simulink model "variable_stiffness_Based_Position"  (R2018b)
settings: Solver=FixedStepAuto  StartTime=0.0  StopTime=1  FixedStep=0.0005  MaxStep=0.002  MinStep=0.001  RelTol=1e-3
model workspace: external: MATLAB File G:\MATLAB\SCARA\SCARA_Robot_DataFile.m (data not in the file)
values from neighbouring files (symbols this model uses):
  Ball = struct    [SCARA_Robot_DataFile.m]
  coff = [1 40 400]    [SCARA_Robot_DataFile.m]
  Plane = struct    [SCARA_Robot_DataFile.m]
  smiData = struct    [SCARA_Robot_DataFile.m]
undefined symbols (not defined in the file or in its folder): sigbuilder_block, X, Y, Z
libraries: sm_lib x81, nesl_utility x44, robotmaniplib x9, Contact_Forces_Lib x3, Parts_Lib x2, cstblocks x1, simulink x1
(part 1 of 2)
settings Model: Creator=wqq  LastModifiedBy=wqq
settings SolverCC: InitialStep=0.001  ZeroCrossAlgorithm=Adaptive
settings DebuggingCC: IgnoredZcDiagnostic=none

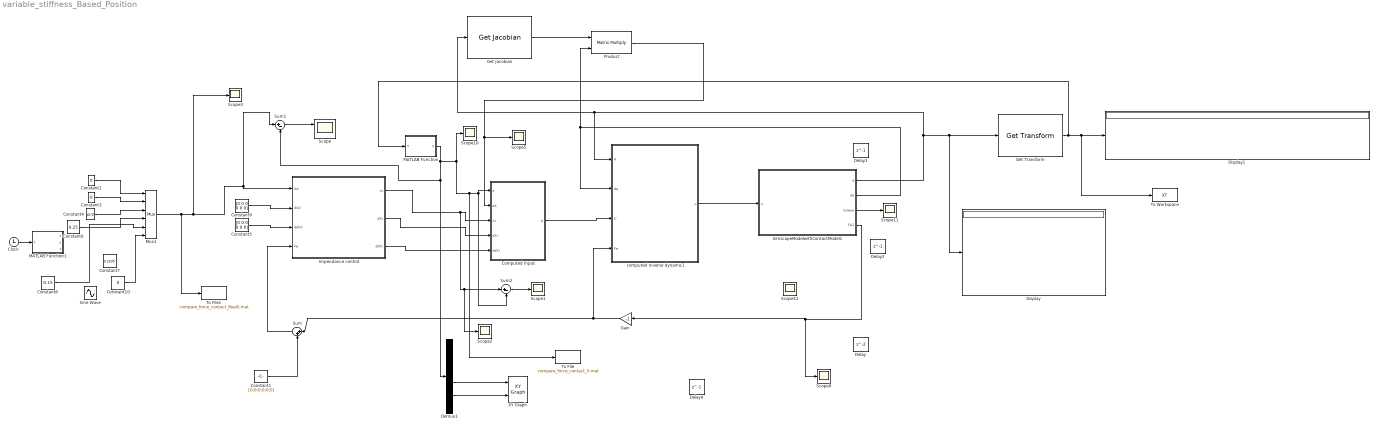
== system variable_stiffness_Based_Position ==
  " Computed Input" : Subsystem
  Clock : Clock
  Constant1 : Constant  Value=[0;0;0;0;0;0]  VectorParams1D=off
  Constant10 : Constant  Value=0
  Constant2 : Constant  Value=0
  Constant3 : Constant  Value=0
  Constant4 : Constant  Value=pi/2
  Constant5 : Constant  Value=[0 0 0 0 0 0]  VectorParams1D=off
  Constant6 : Constant  Value=0.25
  Constant7 : Constant  Value=0.2235
  Constant8 : Constant  Value=0.15
  Constant9 : Constant  Value=[0 0 0 0 0 0]  VectorParams1D=off
  Delay : Delay
  Delay1 : Delay  DelayLength=1  InitialCondition=[0;pi/2;0;0]
  Delay2 : Delay  DelayLength=1  InitialCondition=[0;0;0;0]
  Delay4 : Delay  DelayLength=1  InitialCondition=[0;0;0;0;0;0]
  Demux1 : Demux  Outputs=6
  Display : Display
  Display1 : Display
  Gain : Gain  Gain=-1
  Get Jacobian : robotmaniplib/Get Jacobian  RigidBodyTree=SCARA_Robot  EndEffector=Body5
      settings: SourceProductName=Robotics System Toolbox
  Get Transform : robotmaniplib/Get Transform  RigidBodyTree=SCARA_Robot  SourceBody=Body5  TargetBody=Body7
      settings: SourceProductName=Robotics System Toolbox
  Impendance control : Subsystem
  MATLAB Function : MATLAB Function  TreatAsAtomicUnit=on
  MATLAB Function1 : MATLAB Function  TreatAsAtomicUnit=on
  Mux1 : Mux  Inputs=6
  Product : Product  Multiplication=Matrix(*)
  Scope : Scope  NumInputPorts=2
  Scope{1..3,5,9..12} (8 alike) : Scope
  SimscapeModelwithContactModel1 : Subsystem
      mask Display: image('SCARA_picture.png');
  Sine Wave : Sin  Amplitude=0.5  Bias=0.2235  Frequency=3  SampleTime=0
  Sum : Sum  Inputs=|++
  Sum1 : Sum  Inputs=|+-
  Sum2 : Sum  Inputs=|+-
  To File : ToFile  Filename=compare_force_contact_X.mat  MatrixName=X  SaveFormat=Timeseries
  To File1 : ToFile  Filename=compare_force_contact_RealX.mat  MatrixName=RealX  SaveFormat=Timeseries
  To Workspace : ToWorkspace  VariableName=XT  SaveFormat=Timeseries  SampleTime=-1
  XY Graph : simulink/Sinks/XY Graph  xmin=-0.4  xmax=0.4  ymin=-0.4  ymax=0.4  st=-1
  computed Inverse dynamic1 : Subsystem
  wires:
  SimscapeModelwithContactModel1/3(torque) -> Scope11/1
  Demux1/4 -> XY Graph/1
  Demux1/5 -> XY Graph/2
  Product/1 -> Scope5/1, " Computed Input"/2(dX)
  Get Jacobian/1 -> Product/1
  Constant3/1 -> Mux1/2
  Constant2/1 -> Mux1/1
  " Computed Input"/1(U) -> computed Inverse dynamic1/3(U)
  Clock/1 -> MATLAB Function1/1(t)
  Get Transform/1 -> MATLAB Function/1(T), To Workspace/1, Display1/1
  MATLAB Function/1(X) -> Sum1/2, Demux1/1, Scope10/1, To File/1, " Computed Input"/1(X), Sum2/2
  Constant4/1 -> Mux1/3
  Impendance control/1(Xr) -> Scope2/1, Sum2/1, " Computed Input"/3(Xr)
  Impendance control/2(dXr) -> " Computed Input"/4(dXr)
  Mux1/1 -> To File1/1, Scope3/1, Sum1/1, Impendance control/1(Xd)
  Constant9/1 -> Impendance control/2(dXd)
  Constant5/1 -> Impendance control/3(ddXd)
  Impendance control/3(ddXr) -> " Computed Input"/5(ddXr)
  Sum/1 -> Impendance control/4(Fe)
  Constant1/1 -> Sum/2
  SimscapeModelwithContactModel1/4(Fe1) -> Gain/1, Scope9/1
  SimscapeModelwithContactModel1/2(dq) -> computed Inverse dynamic1/2(dq), Product/2
  SimscapeModelwithContactModel1/1(q) -> Display/1, Get Transform/1, computed Inverse dynamic1/1(q), Get Jacobian/1
  Sum1/1 -> Scope/1
  Sum2/1 -> Scope1/1
  Gain/1 -> computed Inverse dynamic1/4(Fe), Sum/1
  Constant6/1 -> Mux1/4
  Constant8/1 -> Mux1/5
  Constant10/1 -> Mux1/6
  computed Inverse dynamic1/1(u) -> SimscapeModelwithContactModel1/1(u)

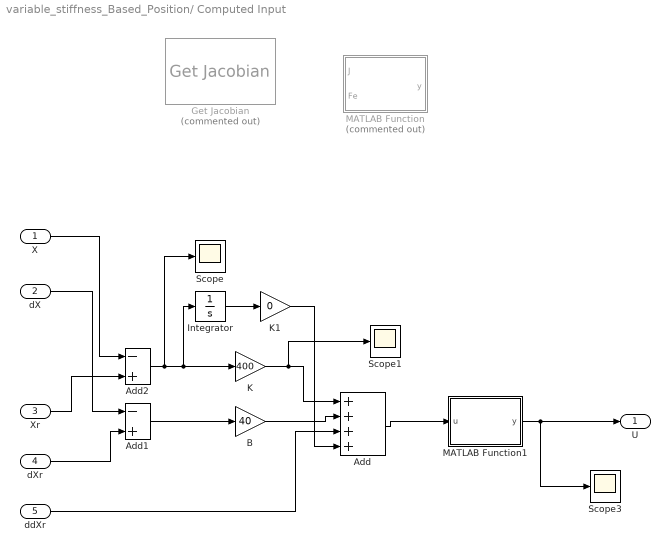
== system variable_stiffness_Based_Position/ Computed Input ==
  X : Inport
  dX : Inport  Port=2
  Xr : Inport  Port=3
  dXr : Inport  Port=4
  ddXr : Inport  Port=5
  Add : Sum  Inputs=++++
  Add1 : Sum  Inputs=-+
  Add2 : Sum  Inputs=-+
  B : Gain  Gain=40
  Get Jacobian : robotmaniplib/Get Jacobian  Commented=on  RigidBodyTree=SCARA_Robot  EndEffector=Body5
      settings: SourceProductName=Robotics System Toolbox
  Integrator : Integrator
  K : Gain  Gain=400
  K1 : Gain  Gain=0
  MATLAB Function : MATLAB Function  Commented=on  TreatAsAtomicUnit=on
  MATLAB Function1 : MATLAB Function  TreatAsAtomicUnit=on
  Scope : Scope
  Scope1 : Scope
  Scope3 : Scope
  U : Outport
  wires:
  ddXr/1 -> Add/3
  dXr/1 -> Add1/2
  dX/1 -> Add1/1
  B/1 -> Add/2
  Xr/1 -> Add2/2
  K/1 -> Scope1/1, Add/1
  Add/1 -> MATLAB Function1/1(u)
  X/1 -> Add2/1
  Add2/1 -> Integrator/1, K/1, Scope/1
  Add1/1 -> B/1
  MATLAB Function1/1(y) -> U/1, Scope3/1
  Integrator/1 -> K1/1
  K1/1 -> Add/4

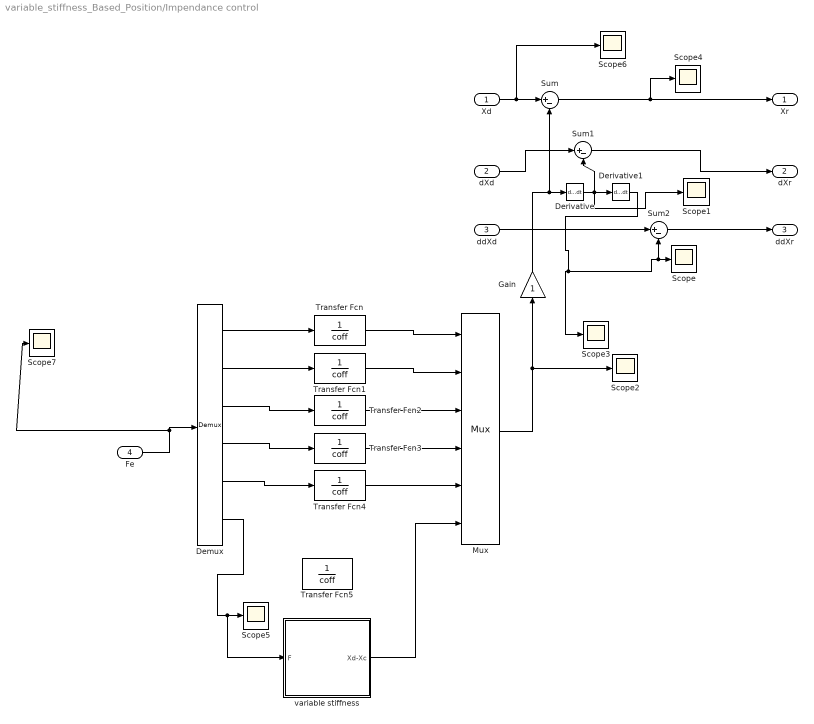
== system variable_stiffness_Based_Position/Impendance control ==
  Xd : Inport
  dXd : Inport  Port=2
  ddXd : Inport  Port=3
  Fe : Inport  Port=4
  Demux : Demux  Outputs=6
  Derivative : Derivative
  Derivative1 : Derivative
  Gain : Gain
  Mux : Mux  Inputs=6
  Scope{,1..7} (8 alike) : Scope
  Sum : Sum  Inputs=|+-
  Sum1 : Sum  Inputs=|+-
  Sum2 : Sum  Inputs=|+-
  Transfer Fcn{,1..5} (6 alike) : TransferFcn  Denominator=coff
  variable stiffness : Subsystem
  Xr : Outport
  dXr : Outport  Port=2
  ddXr : Outport  Port=3
  wires:
  Xd/1 -> Scope6/1, Sum/1
  Sum/1 -> Scope4/1, Xr/1
  dXd/1 -> Sum1/1
  Sum1/1 -> dXr/1
  ddXd/1 -> Sum2/1
  Derivative/1 -> Scope1/1, Derivative1/1, Sum1/2
  Sum2/1 -> ddXr/1
  Demux/1 -> Transfer Fcn/1
  Demux/2 -> Transfer Fcn1/1
  Demux/3 -> Transfer Fcn2/1
  Demux/4 -> Transfer Fcn3/1
  Demux/5 -> Transfer Fcn4/1
  Transfer Fcn4/1 -> Mux/5
  Transfer Fcn3/1 -> Mux/4
  Transfer Fcn2/1 -> Mux/3
  Transfer Fcn1/1 -> Mux/2
  Transfer Fcn/1 -> Mux/1
  Mux/1 -> Scope2/1, Gain/1
  Gain/1 -> Sum/2, Derivative/1
  Fe/1 -> Scope7/1, Demux/1
  Derivative1/1 -> Sum2/2, Scope/1, Scope3/1
  Demux/6 -> variable stiffness/1(F), Scope5/1
  variable stiffness/1(Xd-Xc) -> Mux/6

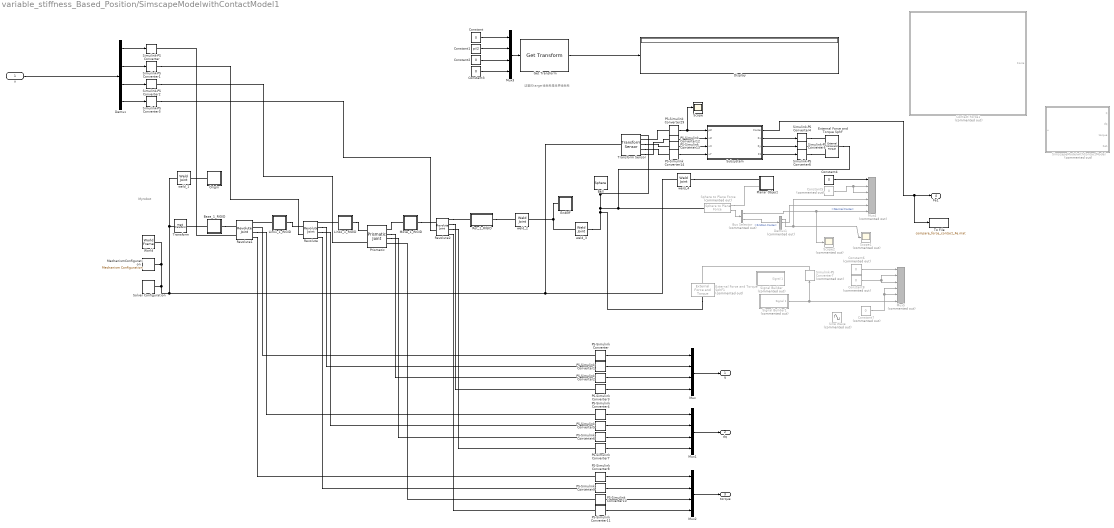
== system variable_stiffness_Based_Position/SimscapeModelwithContactModel1 ==
  note: 这里的target坐标系是世界坐标系
  note: Myrobot
  u : Inport
  Ball : Parts_Lib/Sphere  Tag=CustomStyle  sph_radius=Ball.radius  sph_density=Ball.density  sph_color=red  sph_opacity=1  mark_type=Rings on center planes  arc_width=[40 50]  arc_angle=60  ring_width=5  ring_irad=0.95  mark_color=axes  mark_opacity_x=1  mark_opacity_y=1  mark_opacity_z=1  mark_opacity=1  ring_opacity=0  arc_opacity=0  arc_extr_data=0
  Base_1_RIGID : Subsystem
  Bus Selector : BusSelector  Commented=on  OutputSignals=Normal Force,Friction Force
  Constant{,2..4} (4 alike) : Constant  Value=0
  Constant1 : Constant  Value=pi/2
  Constant{5..8} (4 alike) : Constant  Commented=on  Value=0
  Contact Force1 : Subsystem  Commented=on
  Demux : Demux
  Demux1 : Demux  Commented=on  Outputs=3
  Display : Display
  EndEff : Subsystem
  External Force and Torque SphF : sm_lib/Forces and Torques/External Force and Torque  ForceResolutionFrame=AttachedFrame  EnableForceX=on  EnableForceY=on  EnableForceZ=on  EnableForce=off  TorqueResolutionFrame=AttachedFrame  EnableTorqueX=off  EnableTorqueY=off  EnableTorqueZ=off  EnableTorque=off
  External Force and Torque SphF1 : sm_lib/Forces and Torques/External Force and Torque  Commented=on  ForceResolutionFrame=World  EnableForceX=off  EnableForceY=off  EnableForceZ=on  EnableForce=off  TorqueResolutionFrame=AttachedFrame  EnableTorqueX=off  EnableTorqueY=off  EnableTorqueZ=off  EnableTorque=off
  Get Transform : robotmaniplib/Get Transform  RigidBodyTree=SCARA_Robot  SourceBody=Body5  TargetBody=Body7
      settings: SourceProductName=Robotics System Toolbox
  Link1_1_RIGID : Subsystem
  Link2_1_RIGID : Subsystem
  MechanismConfiguration : sm_lib/Utilities/Mechanism Configuration  UniformGravity=Constant  GravityVector=[0 0 -9.80665]  GravityUnits=m/s^2  LinearizationDelta=0.001
  Move_1_RIGID : Subsystem
  Mux{,1..3} (4 alike) : Mux
  Mux4 : Mux  Commented=on  Inputs=6
  Mux5 : Mux  Commented=on  Inputs=6
  Origin : Subsystem
  PS-Simulink Converter{,1..14,29} (16 alike) : nesl_utility/PS-Simulink Converter  PhysicalDomain=network_engine_domain  SubClassName=ps_output  LeftPortType=input  RightPortType=output  PseudoPeriodic=off  Frequencies=[]  Unit=1  AffineConversion=off
  Planar Object : Subsystem
  Prismatic : sm_lib/Joints/Prismatic Joint  SenseConstraintForce=off  SenseConstraintForceX=off  SenseConstraintForceY=off  SenseConstraintForceZ=off  SenseConstraintTorque=off  SenseConstraintTorqueX=off  SenseConstraintTorqueY=off  SenseConstraintTorqueZ=off  SenseTotalForce=off  SenseTotalForceX=off  SenseTotalForceY=off  SenseTotalForceZ=off  SenseTotalTorque=off  SenseTotalTorqueX=off  SenseTotalTorqueY=off  SenseTotalTorqueZ=off  CompositeWrenchDir=FollowerOnBase  CompositeWrenchFrame=BaseFrame  EquilibriumPosition=0  EquilibriumPositionUnits=m  SpringStiffness=0  SpringStiffnessUnits=N/m  DampingCoefficient=0  DampingCoefficientUnits=N/(m/s)  TorqueActuationMode=InputTorque  MotionActuationMode=ComputedMotion  SensePosition=on  SenseVelocity=on  SenseAcceleration=off  SenseTorqueForce=on  PositionTargetSpecify=on  PositionTargetPriority=High  PositionTargetValue=smiData.PrismaticJoint(1).Pz.Pos  PositionTargetValueUnits=m  VelocityTargetSpecify=off  VelocityTargetPriority=High  VelocityTargetValue=0  VelocityTargetValueUnits=m/s
  Revolute : sm_lib/Joints/Revolute Joint  SenseConstraintForce=off  SenseConstraintForceX=off  SenseConstraintForceY=off  SenseConstraintForceZ=off  SenseConstraintTorque=off  SenseConstraintTorqueX=off  SenseConstraintTorqueY=off  SenseConstraintTorqueZ=off  SenseTotalForce=off  SenseTotalForceX=off  SenseTotalForceY=off  SenseTotalForceZ=off  SenseTotalTorque=off  SenseTotalTorqueX=off  SenseTotalTorqueY=off  SenseTotalTorqueZ=off  CompositeWrenchDir=FollowerOnBase  CompositeWrenchFrame=BaseFrame  EquilibriumPosition=0  EquilibriumPositionUnits=rad  SpringStiffness=0  SpringStiffnessUnits=N*m/rad  DampingCoefficient=0  DampingCoefficientUnits=N*m/(rad/s)  TorqueActuationMode=InputTorque  MotionActuationMode=ComputedMotion  SensePosition=on  SenseVelocity=on  SenseAcceleration=off  SenseTorqueForce=on  PositionTargetSpecify=on  PositionTargetPriority=High  PositionTargetValue=smiData.RevoluteJoint(1).Rz.Pos  PositionTargetValueUnits=deg  VelocityTargetSpecify=off  VelocityTargetPriority=High  VelocityTargetValue=0  VelocityTargetValueUnits=deg/s
  Revolute1 : sm_lib/Joints/Revolute Joint  SenseConstraintForce=off  SenseConstraintForceX=off  SenseConstraintForceY=off  SenseConstraintForceZ=off  SenseConstraintTorque=off  SenseConstraintTorqueX=off  SenseConstraintTorqueY=off  SenseConstraintTorqueZ=off  SenseTotalForce=off  SenseTotalForceX=off  SenseTotalForceY=off  SenseTotalForceZ=off  SenseTotalTorque=off  SenseTotalTorqueX=off  SenseTotalTorqueY=off  SenseTotalTorqueZ=off  CompositeWrenchDir=FollowerOnBase  CompositeWrenchFrame=BaseFrame  EquilibriumPosition=0  EquilibriumPositionUnits=rad  SpringStiffness=0  SpringStiffnessUnits=N*m/rad  DampingCoefficient=0  DampingCoefficientUnits=N*m/(rad/s)  TorqueActuationMode=InputTorque  MotionActuationMode=ComputedMotion  SensePosition=on  SenseVelocity=on  SenseAcceleration=off  SenseTorqueForce=on  PositionTargetSpecify=on  PositionTargetPriority=High  PositionTargetValue=smiData.RevoluteJoint(2).Rz.Pos  PositionTargetValueUnits=deg  VelocityTargetSpecify=off  VelocityTargetPriority=High  VelocityTargetValue=0  VelocityTargetValueUnits=deg/s
  Revolute2 : sm_lib/Joints/Revolute Joint  SenseConstraintForce=off  SenseConstraintForceX=off  SenseConstraintForceY=off  SenseConstraintForceZ=off  SenseConstraintTorque=off  SenseConstraintTorqueX=off  SenseConstraintTorqueY=off  SenseConstraintTorqueZ=off  SenseTotalForce=off  SenseTotalForceX=off  SenseTotalForceY=off  SenseTotalForceZ=off  SenseTotalTorque=off  SenseTotalTorqueX=off  SenseTotalTorqueY=off  SenseTotalTorqueZ=off  CompositeWrenchDir=FollowerOnBase  CompositeWrenchFrame=BaseFrame  EquilibriumPosition=0  EquilibriumPositionUnits=rad  SpringStiffness=0  SpringStiffnessUnits=N*m/rad  DampingCoefficient=0  DampingCoefficientUnits=N*m/(rad/s)  TorqueActuationMode=InputTorque  MotionActuationMode=ComputedMotion  SensePosition=on  SenseVelocity=on  SenseAcceleration=off  SenseTorqueForce=on  PositionTargetSpecify=on  PositionTargetPriority=High  PositionTargetValue=smiData.RevoluteJoint(3).Rz.Pos  PositionTargetValueUnits=deg  VelocityTargetSpecify=off  VelocityTargetPriority=High  VelocityTargetValue=0  VelocityTargetValueUnits=deg/s
  Rot_1_RIGID : Subsystem
  Scope : Scope
  Scope1 : Scope  Commented=on
  Scope2 : Scope  Commented=on
  Signal Builder : Subsystem  Tag=STV Subsys  Commented=on  LoadFcn=sigbuilder_block('load');  StartFcn=sigbuilder_block('start');  StopFcn=sigbuilder_block('stop');  ClipboardFcn=sigbuilder_block('clipboard');  mask(Sigbuilder block){tuvar=[0:10]}
      mask help: Simulink:masks:SigbuilderBlock_MD
      mask init:
      | if ~strcmp(get_param(bdroot(gcbh),'SimulationStatus'),'stopped') tuvar = sigbuilder_block('maskInit'); end
      settings: CopyFcn=sigbuilder_block('copy');  DeleteFcn=sigbuilder_block('delete');  ModelCloseFcn=sigbuilder_block('modelClose');  PreSaveFcn=sigbuilder_block('preSave');  PauseFcn=sigbuilder_block('pause');  ContinueFcn=sigbuilder_block('continue');  NameChangeFcn=sigbuilder_block('namechange');  OpenFcn=sigbuilder_block('open',[437.6 199.2 550.4 400 ]);  CloseFcn=sigbuilder_block('close');
      mask Display: plot(0, 0, 100, 100,[2, 2, 32, 32, 2], [68, 8, 8, 68, 68],[32, 2], [38, 38], [32, 19, 2],[53, 60, 44], [32, 17, 17, 2],[16, 16, 31, 31]);txt = getActiveGroup(gcbh);text(2, 100, txt,'verticalAlignment', 'top');
  Signal Builder1 : Subsystem  Tag=STV Subsys  Commented=on  LoadFcn=sigbuilder_block('load');  StartFcn=sigbuilder_block('start');  StopFcn=sigbuilder_block('stop');  ClipboardFcn=sigbuilder_block('clipboard');  mask(Sigbuilder block){tuvar=[0:10]}
      mask help: Simulink:masks:SigbuilderBlock_MD
      mask init:
      | if ~strcmp(get_param(bdroot(gcbh),'SimulationStatus'),'stopped') tuvar = sigbuilder_block('maskInit'); end
      settings: CopyFcn=sigbuilder_block('copy');  DeleteFcn=sigbuilder_block('delete');  ModelCloseFcn=sigbuilder_block('modelClose');  PreSaveFcn=sigbuilder_block('preSave');  PauseFcn=sigbuilder_block('pause');  ContinueFcn=sigbuilder_block('continue');  NameChangeFcn=sigbuilder_block('namechange');  OpenFcn=sigbuilder_block('open',[437.6 199.2 550.4 400 ]);  CloseFcn=sigbuilder_block('close');
      mask Display: plot(0, 0, 100, 100,[2, 2, 32, 32, 2], [68, 8, 8, 68, 68],[32, 2], [38, 38], [32, 19, 2],[53, 60, 44], [32, 17, 17, 2],[16, 16, 31, 31]);txt = getActiveGroup(gcbh);text(2, 100, txt,'verticalAlignment', 'top');
  SimscapeModelwithContactModel : Subsystem  Commented=on
  Simulink-PS Converter{,1..6} (7 alike) : nesl_utility/Simulink-PS Converter  PhysicalDomain=network_engine_domain  SubClassName=ps_input  LeftPortType=input  RightPortType=output  PseudoPeriodic=off  Frequencies=[]  NoiseDistribution=none  NoiseParameters=[]  Unit=1  AffineConversion=off  FilteringAndDerivatives=provide  SimscapeFilterOrder=1  InputFilterTimeConstant=0.001  UdotUserProvided=0
  Simulink-PS Converter7 : nesl_utility/Simulink-PS Converter  Commented=on  PhysicalDomain=network_engine_domain  SubClassName=ps_input  LeftPortType=input  RightPortType=output  PseudoPeriodic=off  Frequencies=[]  NoiseDistribution=none  NoiseParameters=[]  Unit=1  AffineConversion=off  FilteringAndDerivatives=provide  SimscapeFilterOrder=1  InputFilterTimeConstant=0.001  UdotUserProvided=0
  Sine Wave : Sin  Commented=on  Amplitude=20  SampleTime=0
  Solver Configuration : nesl_utility/Solver Configuration  PhysicalDomain=network_engine_domain  SubClassName=solver  LeftPortType=input  RightPortType=generic  Tones=[]  Harmonics=[]  SimulateNoise=off  Profile=off  UseLocalSampling=off  EnableSwitchedLinearOptims=on  FrequencyDomain=off  UseCCode=off  RelTol=0.001  AbsTol=1e-06  MinStep=1e-09  ToWorkspace=off  RevertToSquareIcSolve=off  NumHomotopyIterations=100  PhasorMode=off  PhasorModeNumHarmonics=1  DoDC=off  ResidualTolerance=1e-09  UseLocalSolver=off  LocalSolverChoice=NE_BACKWARD_EULER_ADVANCER  LocalSolverSampleTime=0.001  DoFixedCost=off  MaxNonlinIter=3  MaxModeIter=2  LinearAlgebra=auto  EquationFormulation=NE_TIME_EF  DelaysMemoryBudget=1024  AutomaticFiltering=on  FilteringTimeConstant=0.001  PartitionStorageMethod=AS_NEEDED  PartitionMemoryBudget=1024
  Sphere to Plane Force : Contact_Forces_Lib/3D/Sphere to Plane Force  Commented=on  sphere_rad=0.03  plane_lenx=1  plane_leny=1  plane_depth=0.1/2  force_law=Linear  k_contact=1e5  b_contact=1e2  pen_full_damp_F=1e-4  pen_exponent=1  custom_param_1=1  custom_param_2=1  friction_law=Stick-Slip Continuous  mu_kinetic=0.5  mu_static=0.7  v_thr=0.001  vis_on=off  vis_opc_en=0  vis_len_plaBz=0.005  vis_clr=[0.9 0.2 0.2]  vis_opc=0.7
  Subsystem : Subsystem
  To File : ToFile  Filename=compare_force_contact_Fe.mat  MatrixName=Fe  SaveFormat=Timeseries
  Transform : sm_lib/Frames and Transforms/Rigid Transform  TranslationMethod=Cartesian  TranslationStandardOffset=0  TranslationLengthUnit=mm  TranslationStandardAxis=+Z  TranslationCartesianOffset=smiData.RigidTransform(9).translation  TranslationROffset=0  TranslationROffsetUnits=m  TranslationZOffset=0  TranslationZOffsetUnits=m  TranslationThetaOffset=0  TranslationThetaOffsetUnits=deg  RotationMethod=ArbitraryAxis  RotationAngleUnits=rad  RotationStandardAxis=+Z  RotationAngle=smiData.RigidTransform(9).angle  RotationArbitraryAxis=smiData.RigidTransform(9).axis  FollAlignAxisA=+X  BaseAlignAxisA=+Y  FollAlignAxisB=+Y  BaseAlignAxisB=+Z  RotationSequenceAxes=FollowerAxes  RotationSequence=XYX  RotationSequenceAngles=[0 0 0]  RotationSequenceAnglesUnits=deg  RotationMatrix=[1 0 0; 0 1 0; 0 0 1]
  Transform Sensor : sm_lib/Frames and Transforms/Transform Sensor  MeasurementFrame=World  SenseAngle=off  SenseAxis=off  SenseAngle1=off  SenseAngle2=off  SenseAngle3=off  SenseQ=off  SenseR=off  SenseOmegaX=off  SenseOmegaY=off  SenseOmegaZ=off  SenseOmega1=off  SenseOmega2=off  SenseOmega3=off  SenseQDot=off  SenseRDot=off  SenseAlphaX=off  SenseAlphaY=off  SenseAlphaZ=off  SenseAlpha1=off  SenseAlpha2=off  SenseAlpha3=off  SenseQDDot=off  SenseRDDot=off  SenseX=off  SenseY=off  SenseZ=on  SenseRad=off  SenseAzim=off  SenseDist=off  SenseInc=off  SenseXDot=on  SenseYDot=on  SenseZDot=on  SenseRadDot=off  SenseAzimDot=off  SenseDistDot=off  SenseIncDot=off  SenseXDDot=off  SenseYDDot=off  SenseZDDot=off  SenseRadDDot=off  SenseAzimDDot=off  SenseDistDDot=off  SenseIncDDot=off
  World : sm_lib/Frames and Transforms/World Frame
  weld_{1..4} (4 alike) : sm_lib/Joints/Weld Joint  SenseConstraintForce=off  SenseConstraintForceX=off  SenseConstraintForceY=off  SenseConstraintForceZ=off  SenseConstraintTorque=off  SenseConstraintTorqueX=off  SenseConstraintTorqueY=off  SenseConstraintTorqueZ=off  SenseTotalForce=off  SenseTotalForceX=off  SenseTotalForceY=off  SenseTotalForceZ=off  SenseTotalTorque=off  SenseTotalTorqueX=off  SenseTotalTorqueY=off  SenseTotalTorqueZ=off  CompositeWrenchDir=FollowerOnBase  CompositeWrenchFrame=BaseFrame
  q : Outport
  dq : Outport  Port=2
  torque : Outport  Port=3
  Fe1 : Outport  Port=4
  wires:
  Demux/4 -> Simulink-PS Converter3/1
  Mux1/1 -> dq/1
  PS-Simulink Converter10/1 -> Mux2/3
  PS-Simulink Converter8/1 -> Mux2/1
  Demux/1 -> Simulink-PS Converter/1
  PS-Simulink Converter11/1 -> Mux2/4
  PS-Simulink Converter5/1 -> Mux1/2
  PS-Simulink Converter/1 -> Mux/1
  Mux2/1 -> torque/1
  PS-Simulink Converter1/1 -> Mux/2
  Demux/2 -> Simulink-PS Converter1/1
  PS-Simulink Converter9/1 -> Mux2/2
  PS-Simulink Converter6/1 -> Mux1/3
  PS-Simulink Converter7/1 -> Mux1/4
  PS-Simulink Converter4/1 -> Mux1/1
  Mux/1 -> q/1
  PS-Simulink Converter2/1 -> Mux/3
  PS-Simulink Converter3/1 -> Mux/4
  Mux3/1 -> Get Transform/1
  Constant/1 -> Mux3/1
  Constant1/1 -> Mux3/2
  Constant2/1 -> Mux3/3
  Constant3/1 -> Mux3/4
  u/1 -> Demux/1
  Get Transform/1 -> Display/1
  Constant4/1 -> Mux4/1
  Constant5/1 -> Mux4/3, Mux4/2
  PS-Simulink Converter29/1 -> Scope/1, Subsystem/1(pZ)
  PS-Simulink Converter12/1 -> Subsystem/2(vZ)
  PS-Simulink Converter14/1 -> Subsystem/4(vY)
  PS-Simulink Converter13/1 -> Subsystem/3(vX)
  Demux/3 -> Simulink-PS Converter2/1
  Sphere to Plane Force/1 -> Bus Selector/1
  Bus Selector/1 -> Scope2/1, Mux4/6  "<Normal Force>"
  Bus Selector/2 -> Demux1/1  "<Friction Force>"
  Demux1/2 -> Mux4/5
  Demux1/1 -> Mux4/4, Scope1/1
  Constant8/1 -> Mux5/2, Mux5/3
  Constant6/1 -> Mux5/1
  Subsystem/2(Fx) -> Simulink-PS Converter4/1
  Subsystem/3(Fy) -> Simulink-PS Converter5/1
  Subsystem/4(Fz) -> Simulink-PS Converter6/1
  Signal Builder1/1(Signal 1) -> Simulink-PS Converter7/1, Mux5/6
  Constant7/1 -> Mux5/5, Mux5/4
  Subsystem/1(Force) -> To File/1, Fe1/1
  connections:
  Revolute2/RConn3 -- PS-Simulink Converter7/LConn1
  Revolute/RConn2 -- PS-Simulink Converter1/LConn1
  Link2_1_RIGID/LConn1 -- Revolute/RConn1
  Move_1_RIGID/LConn1 -- Prismatic/RConn1
  Link1_1_RIGID/LConn1 -- Revolute1/RConn1
  Base_1_RIGID/LConn1 -- Transform/RConn1
  Revolute2/RConn2 -- PS-Simulink Converter3/LConn1
  Revolute1/LConn2 -- Simulink-PS Converter/RConn1
  Revolute1/RConn3 -- PS-Simulink Converter4/LConn1
  Simulink-PS Converter3/RConn1 -- Revolute2/LConn2
  Revolute1/RConn4 -- PS-Simulink Converter8/LConn1
  Move_1_RIGID/RConn1 -- Revolute2/LConn1
  PS-Simulink Converter/LConn1 -- Revolute1/RConn2
  Revolute/RConn4 -- PS-Simulink Converter9/LConn1
  Link2_1_RIGID/RConn1 -- Prismatic/LConn1
  Base_1_RIGID/RConn1 -- Revolute1/LConn1
  Link1_1_RIGID/RConn1 -- Revolute/LConn1
  Revolute2/RConn1 -- Rot_1_RIGID/LConn1
  Prismatic/RConn2 -- PS-Simulink Converter2/LConn1
  Revolute2/RConn4 -- PS-Simulink Converter11/LConn1
  Simulink-PS Converter2/RConn1 -- Prismatic/LConn2
  Simulink-PS Converter1/RConn1 -- Revolute/LConn2
  Revolute/RConn3 -- PS-Simulink Converter5/LConn1
  Prismatic/RConn3 -- PS-Simulink Converter6/LConn1
  Rot_1_RIGID/RConn1 -- weld_2/LConn1
  EndEff/LConn1 -- weld_2/RConn1 -- weld_3/LConn1
  Origin/LConn1 -- weld_1/RConn1
  Ball/LConn1 -- Transform Sensor/RConn1 -- External Force and Torque SphF1/RConn1 -- weld_3/RConn1 -- External Force and Torque SphF/RConn1 -- Sphere to Plane Force/LConn1
  weld_1/LConn1 -- Transform/LConn1 -- World/RConn1 -- MechanismConfiguration/RConn1 -- Solver Configuration/RConn1 -- Transform Sensor/LConn1 -- weld_4/LConn1
  PS-Simulink Converter29/LConn1 -- Transform Sensor/RConn2
  weld_4/RConn1 -- Planar Object/LConn1
  PS-Simulink Converter10/LConn1 -- Prismatic/RConn4
  Transform Sensor/RConn3 -- PS-Simulink Converter13/LConn1
  Transform Sensor/RConn4 -- PS-Simulink Converter14/LConn1
  Transform Sensor/RConn5 -- PS-Simulink Converter12/LConn1
  Sphere to Plane Force/RConn1 -- Planar Object/LConn2
  Simulink-PS Converter4/RConn1 -- External Force and Torque SphF/LConn1
  Simulink-PS Converter5/RConn1 -- External Force and Torque SphF/LConn2
  Simulink-PS Converter6/RConn1 -- External Force and Torque SphF/LConn3
  Simulink-PS Converter7/RConn1 -- External Force and Torque SphF1/LConn1

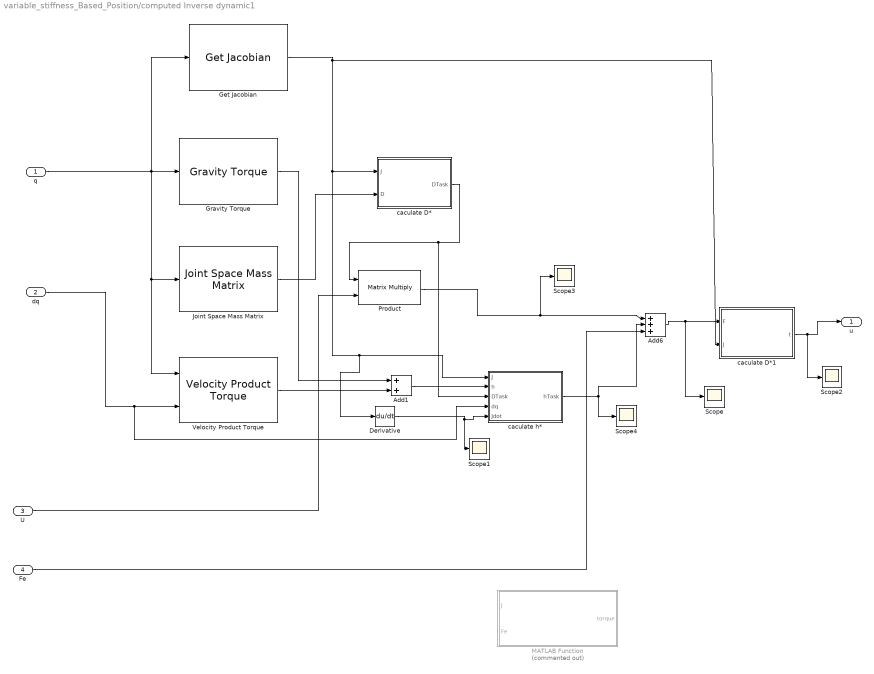
== system variable_stiffness_Based_Position/computed Inverse dynamic1 ==
  q : Inport
  dq : Inport  Port=2
  U : Inport  Port=3
  Fe : Inport  Port=4
  Add1 : Sum
  Add6 : Sum  Inputs=+++
  Derivative : Derivative
  Get Jacobian : robotmaniplib/Get Jacobian  RigidBodyTree=SCARA_Robot  EndEffector=Body5
      settings: SourceProductName=Robotics System Toolbox
  Gravity Torque : robotmaniplib/Gravity Torque  RigidBodyTree=SCARA_Robot
      settings: SourceProductName=Robotics System Toolbox
  Joint Space Mass Matrix : robotmaniplib/Joint Space Mass Matrix  RigidBodyTree=SCARA_Robot
      settings: SourceProductName=Robotics System Toolbox
  MATLAB Function : MATLAB Function  Commented=on  TreatAsAtomicUnit=on
  Product : Product  Multiplication=Matrix(*)
  Scope{,1..4} (5 alike) : Scope
  Velocity Product Torque : robotmaniplib/Velocity Product Torque  RigidBodyTree=SCARA_Robot
      settings: SourceProductName=Robotics System Toolbox
  caculate D* : MATLAB Function  TreatAsAtomicUnit=on
  caculate D*1 : MATLAB Function  TreatAsAtomicUnit=on
  caculate h* : MATLAB Function  TreatAsAtomicUnit=on
  u : Outport
  wires:
  q/1 -> Velocity Product Torque/1, Joint Space Mass Matrix/1, Get Jacobian/1, Gravity Torque/1
  Velocity Product Torque/1 -> Add1/2
  U/1 -> Product/2
  Joint Space Mass Matrix/1 -> caculate D*/2(D)
  Get Jacobian/1 -> Derivative/1, caculate h*/1(J), caculate D*/1(J), caculate D*1/2(J)
  caculate D*/1(DTask) -> caculate h*/3(DTask), Product/1
  Product/1 -> Scope3/1, Add6/1
  Gravity Torque/1 -> Add1/1
  Add1/1 -> caculate h*/2(h)
  dq/1 -> caculate h*/4(dq), Velocity Product Torque/2
  caculate D*1/1(t) -> Scope2/1, u/1
  Add6/1 -> Scope/1, caculate D*1/1(F)
  Derivative/1 -> Scope1/1, caculate h*/5(Jdot)
  caculate h*/1(hTask) -> Add6/2, Scope4/1
  Fe/1 -> Add6/3

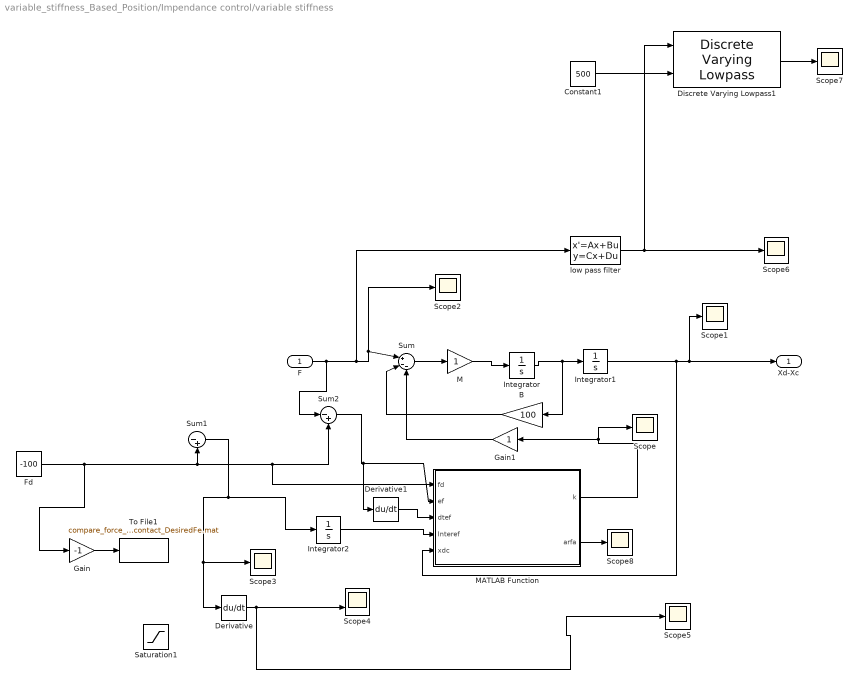
== system variable_stiffness_Based_Position/Impendance control/variable stiffness ==
  F : Inport
  B : Gain  Gain=100
  Constant1 : Constant  Value=500
  Derivative : Derivative
  Derivative1 : Derivative
  Discrete Varying Lowpass1 : cstblocks/Linear Parameter Varying/Discrete Varying Lowpass  N=1  w0=100  Ts=0.0005
      settings: SourceProductName=Control System Toolbox  SourceProductBaseCode=CT
  Fd : Constant  Value=-100
  Gain : Gain  Gain=-1
  Gain1 : Gain
  Integrator : Integrator  InitialCondition=0.0001  UpperSaturationLimit=1000  LowerSaturationLimit=-1000  IgnoreLimit=on
  Integrator1 : Integrator  InitialCondition=0.001
  Integrator2 : Integrator  UpperSaturationLimit=1000  LowerSaturationLimit=-1000  IgnoreLimit=on
  M : Gain
  MATLAB Function : MATLAB Function  TreatAsAtomicUnit=on
  Saturation1 : Saturate  UpperLimit=1000  LowerLimit=-1000
  Scope{,1..3,5..8} (8 alike) : Scope
  Scope4 : Scope  NumInputPorts=2
  Sum : Sum  Inputs=|+--
  Sum1 : Sum  Inputs=|-+
  Sum2 : Sum  Inputs=|-+
  To File1 : ToFile  Filename=compare_force_contact_DesiredFe.mat  MatrixName=DesiredFe  SaveFormat=Timeseries
  low pass filter : StateSpace  A=-100*eye(1)  B=100*eye(1)  C=eye(1)  D=zeros(1,1)  InitialCondition=zeros(1,1)
  Xd-Xc : Outport
  wires:
  Integrator/1 -> B/1, Integrator1/1
  F/1 -> Sum2/1, low pass filter/1, Scope2/1, Sum/1
  Sum/1 -> M/1
  B/1 -> Sum/2
  M/1 -> Integrator/1
  Gain1/1 -> Sum/3
  low pass filter/1 -> Discrete Varying Lowpass1/1, Scope6/1
  Integrator2/1 -> MATLAB Function/4(Interef)
  Sum1/1 -> Integrator2/1, Derivative/1, Scope3/1
  Discrete Varying Lowpass1/1 -> Scope7/1
  Constant1/1 -> Discrete Varying Lowpass1/2
  MATLAB Function/1(k) -> Gain1/1, Scope/1
  Integrator1/1 -> MATLAB Function/5(xdc), Xd-Xc/1, Scope1/1
  Derivative/1 -> Scope5/1, Scope4/2
  Gain/1 -> To File1/1
  Fd/1 -> Gain/1, MATLAB Function/1(fd), Sum2/2, Sum1/2
  MATLAB Function/2(arfa) -> Scope8/1
  Sum2/1 -> Derivative1/1, MATLAB Function/2(ef)
  Derivative1/1 -> MATLAB Function/3(dtef)

== system variable_stiffness_Based_Position/SimscapeModelwithContactModel1/Base_1_RIGID ==
  ReferenceFrame : sm_lib/Frames and Transforms/Reference Frame
  Solid : sm_lib/Body Elements/Solid  InertiaType=Custom  Mass=smiData.Solid(3).mass  MassUnits=kg  CenterOfMass=smiData.Solid(3).CoM  CenterOfMassUnits=mm  MomentsOfInertia=smiData.Solid(3).MoI  MomentsOfInertiaUnits=kg*mm^2  ProductsOfInertia=smiData.Solid(3).PoI  ProductsOfInertiaUnits=kg*mm^2  BasedOnType=Density  Density=1000  DensityUnits=kg/m^3  DoExposeReferenceFrame=off  SerializedFrames=<Frames><Frame><Id>Frame1</Id><Value><Name>F2</Name><Origin><Source>GeometricFeature</Source><FeatureName>cylindrical surface 2</FeatureName></Origin><PrimaryAxis><DefinedDirection>+Z</DefinedDirection><Source>ReferenceFrame</Source><SourceDirection>+Z</SourceDirection><FeatureName></FeatureName></PrimaryAxis><SecondaryAxis><DefinedDirection>+X</DefinedDirection><Source>ReferenceFrame</Source><SourceDirection>+X</SourceDirection><FeatureName></FeatureName></SecondaryAxis></Value></Frame></Frames>  GraphicType=FromGeometry  MarkerShape=Sphere  MarkerSize=10  GraphicVisPropType=SimpleVisualProperties  GraphicDiffuseColor=smiData.Solid(3).color  GraphicSpecularColor=[0.5 0.5 0.5 1.0]  GraphicAmbientColor=[0.15 0.15 0.15 1.0]  GraphicEmissiveColor=[0.0 0.0 0.0 1.0]  GraphicShininess=75  GraphicOpacity=smiData.Solid(3).opacity  GeometryShape=FromFile  RectangleSize=[1 1]  RectangleSizeUnits=m  BrickDimensions=[1 1 1]  BrickDimensionUnits=m  CylinderRadius=1  CylinderRadiusUnits=m  CylinderLength=1  CylinderLengthUnits=m  SphereRadius=1  SphereRadiusUnits=m  EllipsoidRadii=[1 1 1]  EllipsoidRadiiUnits=m  ExtrusionCrossSection=[1 1; -1 1; -1 -1; 1 -1]  ExtrusionCrossSectionUnits=m  ExtrusionLength=1  ExtrusionLengthUnits=m  PolygonNumSides=3  PolygonOuterRadius=1  PolygonOuterRadiusUnits=m  ExtGeomFileType=STEP  ExtGeomFileName=Base_默认_sldprt.STEP  ExtGeomFileUnits=m  RevolutionCrossSection=[1 1; 1 -1; 2 -1; 2 1]  RevolutionCrossSectionUnits=m  RevolutionExtent=Full  RevolutionAngle=180  RevolutionAngleUnits=deg
  Transform : sm_lib/Frames and Transforms/Rigid Transform  TranslationMethod=Cartesian  TranslationStandardOffset=0  TranslationLengthUnit=mm  TranslationStandardAxis=+Z  TranslationCartesianOffset=smiData.RigidTransform(3).translation  TranslationROffset=0  TranslationROffsetUnits=m  TranslationZOffset=0  TranslationZOffsetUnits=m  TranslationThetaOffset=0  TranslationThetaOffsetUnits=deg  RotationMethod=ArbitraryAxis  RotationAngleUnits=rad  RotationStandardAxis=+Z  RotationAngle=smiData.RigidTransform(3).angle  RotationArbitraryAxis=smiData.RigidTransform(3).axis  FollAlignAxisA=+X  BaseAlignAxisA=+Y  FollAlignAxisB=+Y  BaseAlignAxisB=+Z  RotationSequenceAxes=FollowerAxes  RotationSequence=XYX  RotationSequenceAngles=[0 0 0]  RotationSequenceAnglesUnits=deg  RotationMatrix=[1 0 0; 0 1 0; 0 0 1]
  F1 : PMIOPort  Side=Left
  F : PMIOPort  Port=2  Side=Right
  connections:
  ReferenceFrame/RConn1 -- Solid/LConn1 -- Transform/LConn1 -- F1/RConn1
  Transform/RConn1 -- F/RConn1

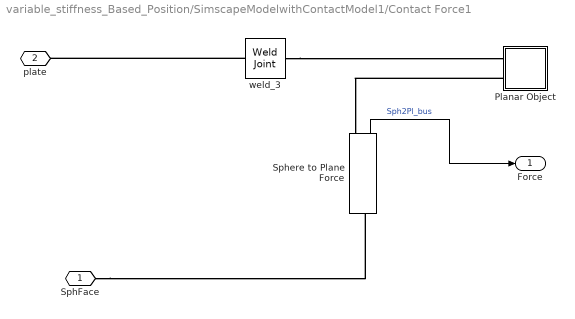
== system variable_stiffness_Based_Position/SimscapeModelwithContactModel1/Contact Force1 ==
  Planar Object : Subsystem
  Sphere to Plane Force : Contact_Forces_Lib/3D/Sphere to Plane Force  sphere_rad=Ball.radius  plane_lenx=Plane.width  plane_leny=Plane.length  plane_depth=0.1/2  force_law=Nonlinear  k_contact=1e7  b_contact=1e3  pen_full_damp_F=1e-4  pen_exponent=1  custom_param_1=1  custom_param_2=1  friction_law=None  mu_kinetic=0.5  mu_static=0.7  v_thr=0.001  vis_on=off  vis_opc_en=0  vis_len_plaBz=Plane.depth*0.1  vis_clr=[0.9 0.2 0.2]  vis_opc=0.7
  weld_3 : sm_lib/Joints/Weld Joint  SenseConstraintForce=off  SenseConstraintForceX=off  SenseConstraintForceY=off  SenseConstraintForceZ=off  SenseConstraintTorque=off  SenseConstraintTorqueX=off  SenseConstraintTorqueY=off  SenseConstraintTorqueZ=off  SenseTotalForce=off  SenseTotalForceX=off  SenseTotalForceY=off  SenseTotalForceZ=off  SenseTotalTorque=off  SenseTotalTorqueX=off  SenseTotalTorqueY=off  SenseTotalTorqueZ=off  CompositeWrenchDir=FollowerOnBase  CompositeWrenchFrame=BaseFrame
  SphFace : PMIOPort  Side=Left
  plate : PMIOPort  Port=2  Side=Left
  Force : Outport
  wires:
  Sphere to Plane Force/1 -> Force/1  "Sph2Pl_bus"
  connections:
  weld_3/RConn1 -- Planar Object/LConn1
  SphFace/RConn1 -- Sphere to Plane Force/LConn1
  weld_3/LConn1 -- plate/RConn1
  Planar Object/LConn2 -- Sphere to Plane Force/RConn1

== system variable_stiffness_Based_Position/SimscapeModelwithContactModel1/EndEff ==
  ReferenceFrame : sm_lib/Frames and Transforms/Reference Frame
  F : PMIOPort  Side=Left
  connections:
  ReferenceFrame/RConn1 -- F/RConn1

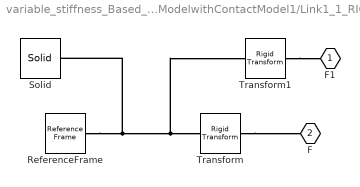
== system variable_stiffness_Based_Position/SimscapeModelwithContactModel1/Link1_1_RIGID ==
  ReferenceFrame : sm_lib/Frames and Transforms/Reference Frame
  Solid : sm_lib/Body Elements/Solid  InertiaType=Custom  Mass=smiData.Solid(4).mass  MassUnits=kg  CenterOfMass=smiData.Solid(4).CoM  CenterOfMassUnits=mm  MomentsOfInertia=smiData.Solid(4).MoI  MomentsOfInertiaUnits=kg*mm^2  ProductsOfInertia=smiData.Solid(4).PoI  ProductsOfInertiaUnits=kg*mm^2  BasedOnType=Density  Density=1000  DensityUnits=kg/m^3  DoExposeReferenceFrame=on  SerializedFrames=<Frames/>  GraphicType=FromGeometry  MarkerShape=Sphere  MarkerSize=10  GraphicVisPropType=SimpleVisualProperties  GraphicDiffuseColor=smiData.Solid(4).color  GraphicSpecularColor=[0.5 0.5 0.5 1.0]  GraphicAmbientColor=[0.15 0.15 0.15 1.0]  GraphicEmissiveColor=[0.0 0.0 0.0 1.0]  GraphicShininess=75  GraphicOpacity=smiData.Solid(4).opacity  GeometryShape=FromFile  RectangleSize=[1 1]  RectangleSizeUnits=m  BrickDimensions=[1 1 1]  BrickDimensionUnits=m  CylinderRadius=1  CylinderRadiusUnits=m  CylinderLength=1  CylinderLengthUnits=m  SphereRadius=1  SphereRadiusUnits=m  EllipsoidRadii=[1 1 1]  EllipsoidRadiiUnits=m  ExtrusionCrossSection=[1 1; -1 1; -1 -1; 1 -1]  ExtrusionCrossSectionUnits=m  ExtrusionLength=1  ExtrusionLengthUnits=m  PolygonNumSides=3  PolygonOuterRadius=1  PolygonOuterRadiusUnits=m  ExtGeomFileType=STEP  ExtGeomFileName=Link1_默认_sldprt.STEP  ExtGeomFileUnits=m  RevolutionCrossSection=[1 1; 1 -1; 2 -1; 2 1]  RevolutionCrossSectionUnits=m  RevolutionExtent=Full  RevolutionAngle=180  RevolutionAngleUnits=deg
  Transform : sm_lib/Frames and Transforms/Rigid Transform  TranslationMethod=Cartesian  TranslationStandardOffset=0  TranslationLengthUnit=mm  TranslationStandardAxis=+Z  TranslationCartesianOffset=smiData.RigidTransform(1).translation  TranslationROffset=0  TranslationROffsetUnits=m  TranslationZOffset=0  TranslationZOffsetUnits=m  TranslationThetaOffset=0  TranslationThetaOffsetUnits=deg  RotationMethod=ArbitraryAxis  RotationAngleUnits=rad  RotationStandardAxis=+Z  RotationAngle=smiData.RigidTransform(1).angle  RotationArbitraryAxis=smiData.RigidTransform(1).axis  FollAlignAxisA=+X  BaseAlignAxisA=+Y  FollAlignAxisB=+Y  BaseAlignAxisB=+Z  RotationSequenceAxes=FollowerAxes  RotationSequence=XYX  RotationSequenceAngles=[0 0 0]  RotationSequenceAnglesUnits=deg  RotationMatrix=[1 0 0; 0 1 0; 0 0 1]
  Transform1 : sm_lib/Frames and Transforms/Rigid Transform  TranslationMethod=Cartesian  TranslationStandardOffset=0  TranslationLengthUnit=mm  TranslationStandardAxis=+Z  TranslationCartesianOffset=smiData.RigidTransform(4).translation  TranslationROffset=0  TranslationROffsetUnits=m  TranslationZOffset=0  TranslationZOffsetUnits=m  TranslationThetaOffset=0  TranslationThetaOffsetUnits=deg  RotationMethod=ArbitraryAxis  RotationAngleUnits=rad  RotationStandardAxis=+Z  RotationAngle=smiData.RigidTransform(4).angle  RotationArbitraryAxis=smiData.RigidTransform(4).axis  FollAlignAxisA=+X  BaseAlignAxisA=+Y  FollAlignAxisB=+Y  BaseAlignAxisB=+Z  RotationSequenceAxes=FollowerAxes  RotationSequence=XYX  RotationSequenceAngles=[0 0 0]  RotationSequenceAnglesUnits=deg  RotationMatrix=[1 0 0; 0 1 0; 0 0 1]
  F1 : PMIOPort  Side=Left
  F : PMIOPort  Port=2  Side=Right
  connections:
  Solid/RConn1 -- Transform/LConn1 -- Transform1/LConn1 -- ReferenceFrame/RConn1
  Transform/RConn1 -- F/RConn1
  Transform1/RConn1 -- F1/RConn1

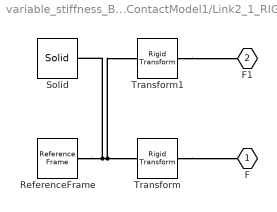
== system variable_stiffness_Based_Position/SimscapeModelwithContactModel1/Link2_1_RIGID ==
  ReferenceFrame : sm_lib/Frames and Transforms/Reference Frame
  Solid : sm_lib/Body Elements/Solid  InertiaType=Custom  Mass=smiData.Solid(1).mass  MassUnits=kg  CenterOfMass=smiData.Solid(1).CoM  CenterOfMassUnits=mm  MomentsOfInertia=smiData.Solid(1).MoI  MomentsOfInertiaUnits=kg*mm^2  ProductsOfInertia=smiData.Solid(1).PoI  ProductsOfInertiaUnits=kg*mm^2  BasedOnType=Density  Density=1000  DensityUnits=kg/m^3  DoExposeReferenceFrame=on  SerializedFrames=<Frames/>  GraphicType=FromGeometry  MarkerShape=Sphere  MarkerSize=10  GraphicVisPropType=SimpleVisualProperties  GraphicDiffuseColor=smiData.Solid(1).color  GraphicSpecularColor=[0.5 0.5 0.5 1.0]  GraphicAmbientColor=[0.15 0.15 0.15 1.0]  GraphicEmissiveColor=[0.0 0.0 0.0 1.0]  GraphicShininess=75  GraphicOpacity=smiData.Solid(1).opacity  GeometryShape=FromFile  RectangleSize=[1 1]  RectangleSizeUnits=m  BrickDimensions=[1 1 1]  BrickDimensionUnits=m  CylinderRadius=1  CylinderRadiusUnits=m  CylinderLength=1  CylinderLengthUnits=m  SphereRadius=1  SphereRadiusUnits=m  EllipsoidRadii=[1 1 1]  EllipsoidRadiiUnits=m  ExtrusionCrossSection=[1 1; -1 1; -1 -1; 1 -1]  ExtrusionCrossSectionUnits=m  ExtrusionLength=1  ExtrusionLengthUnits=m  PolygonNumSides=3  PolygonOuterRadius=1  PolygonOuterRadiusUnits=m  ExtGeomFileType=STEP  ExtGeomFileName=Link2_默认_sldprt.STEP  ExtGeomFileUnits=m  RevolutionCrossSection=[1 1; 1 -1; 2 -1; 2 1]  RevolutionCrossSectionUnits=m  RevolutionExtent=Full  RevolutionAngle=180  RevolutionAngleUnits=deg
  Transform : sm_lib/Frames and Transforms/Rigid Transform  TranslationMethod=Cartesian  TranslationStandardOffset=0  TranslationLengthUnit=mm  TranslationStandardAxis=+Z  TranslationCartesianOffset=smiData.RigidTransform(2).translation  TranslationROffset=0  TranslationROffsetUnits=m  TranslationZOffset=0  TranslationZOffsetUnits=m  TranslationThetaOffset=0  TranslationThetaOffsetUnits=deg  RotationMethod=ArbitraryAxis  RotationAngleUnits=rad  RotationStandardAxis=+Z  RotationAngle=smiData.RigidTransform(2).angle  RotationArbitraryAxis=smiData.RigidTransform(2).axis  FollAlignAxisA=+X  BaseAlignAxisA=+Y  FollAlignAxisB=+Y  BaseAlignAxisB=+Z  RotationSequenceAxes=FollowerAxes  RotationSequence=XYX  RotationSequenceAngles=[0 0 0]  RotationSequenceAnglesUnits=deg  RotationMatrix=[1 0 0; 0 1 0; 0 0 1]
  Transform1 : sm_lib/Frames and Transforms/Rigid Transform  TranslationMethod=Cartesian  TranslationStandardOffset=0  TranslationLengthUnit=mm  TranslationStandardAxis=+Z  TranslationCartesianOffset=smiData.RigidTransform(5).translation  TranslationROffset=0  TranslationROffsetUnits=m  TranslationZOffset=0  TranslationZOffsetUnits=m  TranslationThetaOffset=0  TranslationThetaOffsetUnits=deg  RotationMethod=ArbitraryAxis  RotationAngleUnits=rad  RotationStandardAxis=+Z  RotationAngle=smiData.RigidTransform(5).angle  RotationArbitraryAxis=smiData.RigidTransform(5).axis  FollAlignAxisA=+X  BaseAlignAxisA=+Y  FollAlignAxisB=+Y  BaseAlignAxisB=+Z  RotationSequenceAxes=FollowerAxes  RotationSequence=XYX  RotationSequenceAngles=[0 0 0]  RotationSequenceAnglesUnits=deg  RotationMatrix=[1 0 0; 0 1 0; 0 0 1]
  F : PMIOPort  Side=Left
  F1 : PMIOPort  Port=2  Side=Right
  connections:
  Solid/RConn1 -- ReferenceFrame/RConn1 -- Transform/LConn1 -- Transform1/LConn1
  Transform/RConn1 -- F/RConn1
  Transform1/RConn1 -- F1/RConn1

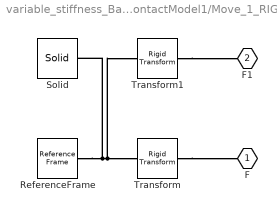
== system variable_stiffness_Based_Position/SimscapeModelwithContactModel1/Move_1_RIGID ==
  ReferenceFrame : sm_lib/Frames and Transforms/Reference Frame
  Solid : sm_lib/Body Elements/Solid  InertiaType=Custom  Mass=smiData.Solid(5).mass  MassUnits=kg  CenterOfMass=smiData.Solid(5).CoM  CenterOfMassUnits=mm  MomentsOfInertia=smiData.Solid(5).MoI  MomentsOfInertiaUnits=kg*mm^2  ProductsOfInertia=smiData.Solid(5).PoI  ProductsOfInertiaUnits=kg*mm^2  BasedOnType=Density  Density=1000  DensityUnits=kg/m^3  DoExposeReferenceFrame=on  SerializedFrames=<Frames/>  GraphicType=FromGeometry  MarkerShape=Sphere  MarkerSize=10  GraphicVisPropType=SimpleVisualProperties  GraphicDiffuseColor=smiData.Solid(5).color  GraphicSpecularColor=[0.5 0.5 0.5 1.0]  GraphicAmbientColor=[0.15 0.15 0.15 1.0]  GraphicEmissiveColor=[0.0 0.0 0.0 1.0]  GraphicShininess=75  GraphicOpacity=smiData.Solid(5).opacity  GeometryShape=FromFile  RectangleSize=[1 1]  RectangleSizeUnits=m  BrickDimensions=[1 1 1]  BrickDimensionUnits=m  CylinderRadius=1  CylinderRadiusUnits=m  CylinderLength=1  CylinderLengthUnits=m  SphereRadius=1  SphereRadiusUnits=m  EllipsoidRadii=[1 1 1]  EllipsoidRadiiUnits=m  ExtrusionCrossSection=[1 1; -1 1; -1 -1; 1 -1]  ExtrusionCrossSectionUnits=m  ExtrusionLength=1  ExtrusionLengthUnits=m  PolygonNumSides=3  PolygonOuterRadius=1  PolygonOuterRadiusUnits=m  ExtGeomFileType=STEP  ExtGeomFileName=Move_默认_sldprt.STEP  ExtGeomFileUnits=m  RevolutionCrossSection=[1 1; 1 -1; 2 -1; 2 1]  RevolutionCrossSectionUnits=m  RevolutionExtent=Full  RevolutionAngle=180  RevolutionAngleUnits=deg
  Transform : sm_lib/Frames and Transforms/Rigid Transform  TranslationMethod=Cartesian  TranslationStandardOffset=0  TranslationLengthUnit=mm  TranslationStandardAxis=+Z  TranslationCartesianOffset=smiData.RigidTransform(6).translation  TranslationROffset=0  TranslationROffsetUnits=m  TranslationZOffset=0  TranslationZOffsetUnits=m  TranslationThetaOffset=0  TranslationThetaOffsetUnits=deg  RotationMethod=ArbitraryAxis  RotationAngleUnits=rad  RotationStandardAxis=+Z  RotationAngle=smiData.RigidTransform(6).angle  RotationArbitraryAxis=smiData.RigidTransform(6).axis  FollAlignAxisA=+X  BaseAlignAxisA=+Y  FollAlignAxisB=+Y  BaseAlignAxisB=+Z  RotationSequenceAxes=FollowerAxes  RotationSequence=XYX  RotationSequenceAngles=[0 0 0]  RotationSequenceAnglesUnits=deg  RotationMatrix=[1 0 0; 0 1 0; 0 0 1]
  Transform1 : sm_lib/Frames and Transforms/Rigid Transform  TranslationMethod=Cartesian  TranslationStandardOffset=0  TranslationLengthUnit=mm  TranslationStandardAxis=+Z  TranslationCartesianOffset=smiData.RigidTransform(7).translation  TranslationROffset=0  TranslationROffsetUnits=m  TranslationZOffset=0  TranslationZOffsetUnits=m  TranslationThetaOffset=0  TranslationThetaOffsetUnits=deg  RotationMethod=ArbitraryAxis  RotationAngleUnits=rad  RotationStandardAxis=+Z  RotationAngle=0  RotationArbitraryAxis=[0 0 1]  FollAlignAxisA=+X  BaseAlignAxisA=+Y  FollAlignAxisB=+Y  BaseAlignAxisB=+Z  RotationSequenceAxes=FollowerAxes  RotationSequence=XYX  RotationSequenceAngles=[0 0 0]  RotationSequenceAnglesUnits=deg  RotationMatrix=[1 0 0; 0 1 0; 0 0 1]
  F : PMIOPort  Side=Left
  F1 : PMIOPort  Port=2  Side=Right
  connections:
  Solid/RConn1 -- ReferenceFrame/RConn1 -- Transform/LConn1 -- Transform1/LConn1
  Transform/RConn1 -- F/RConn1
  Transform1/RConn1 -- F1/RConn1

== system variable_stiffness_Based_Position/SimscapeModelwithContactModel1/Origin ==
  ReferenceFrame : sm_lib/Frames and Transforms/Reference Frame
  F : PMIOPort  Side=Left
  connections:
  ReferenceFrame/RConn1 -- F/RConn1

== system variable_stiffness_Based_Position/SimscapeModelwithContactModel1/Planar Object ==
  Inertia : sm_lib/Body Elements/Solid  InertiaType=Custom  Mass=1e8  MassUnits=kg  CenterOfMass=[0, 0, 0]  CenterOfMassUnits=m  MomentsOfInertia=[1e-08, 1e-08, 1e-08]  MomentsOfInertiaUnits=kg*m^2  ProductsOfInertia=[1e-08, 1e-08, 1e-08]  ProductsOfInertiaUnits=kg*m^2  BasedOnType=Density  Density=1000  DensityUnits=kg/m^3  DoExposeReferenceFrame=on  SerializedFrames=<Frames/>  GraphicType=FromGeometry  MarkerShape=Sphere  MarkerSize=10  GraphicVisPropType=SimpleVisualProperties  GraphicDiffuseColor=[0.5 0.5 0.5]  GraphicSpecularColor=[0.5 0.5 0.5 1.0]  GraphicAmbientColor=[0.15 0.15 0.15 1.0]  GraphicEmissiveColor=[0.0 0.0 0.0 1.0]  GraphicShininess=75  GraphicOpacity=1  GeometryShape=Brick  RectangleSize=[1 1]  RectangleSizeUnits=m  BrickDimensions=[0.1 1 1]  BrickDimensionUnits=m  CylinderRadius=1  CylinderRadiusUnits=m  CylinderLength=1  CylinderLengthUnits=m  SphereRadius=1  SphereRadiusUnits=m  EllipsoidRadii=[1 1 1]  EllipsoidRadiiUnits=m  ExtrusionCrossSection=[1 1; -1 1; -1 -1; 1 -1]  ExtrusionCrossSectionUnits=m  ExtrusionLength=1  ExtrusionLengthUnits=m  PolygonNumSides=3  PolygonOuterRadius=1  PolygonOuterRadiusUnits=m  ExtGeomFileType=STEP  ExtGeomFileUnits=m  RevolutionCrossSection=[1 1; 1 -1; 2 -1; 2 1]  RevolutionCrossSectionUnits=m  RevolutionExtent=Full  RevolutionAngle=180  RevolutionAngleUnits=deg
  InertiaOriginTransform : sm_lib/Frames and Transforms/Rigid Transform  TranslationMethod=Cartesian  TranslationStandardOffset=0  TranslationLengthUnit=m  TranslationStandardAxis=+Z  TranslationCartesianOffset=[0.3, 0, -0.05]  TranslationROffset=0  TranslationROffsetUnits=m  TranslationZOffset=0  TranslationZOffsetUnits=m  TranslationThetaOffset=0  TranslationThetaOffsetUnits=deg  RotationMethod=StandardAxis  RotationAngleUnits=deg  RotationStandardAxis=+Y  RotationAngle=90  RotationArbitraryAxis=[0 0 1]  FollAlignAxisA=+X  BaseAlignAxisA=+Y  FollAlignAxisB=+Y  BaseAlignAxisB=+Z  RotationSequenceAxes=BaseAxes  RotationSequence=XYZ  RotationSequenceAngles=[0, -1, 0]  RotationSequenceAnglesUnits=rad  RotationMatrix=[1 0 0; 0 -1 0; 0 0 -1]
  InertiaOriginTransform1 : sm_lib/Frames and Transforms/Rigid Transform  TranslationMethod=None  TranslationStandardOffset=0  TranslationLengthUnit=m  TranslationStandardAxis=+Z  TranslationCartesianOffset=[0.3, 0, -0.05]  TranslationROffset=0  TranslationROffsetUnits=m  TranslationZOffset=0  TranslationZOffsetUnits=m  TranslationThetaOffset=0  TranslationThetaOffsetUnits=deg  RotationMethod=RotationMatrix  RotationAngleUnits=deg  RotationStandardAxis=+Y  RotationAngle=90  RotationArbitraryAxis=[0 0 1]  FollAlignAxisA=+X  BaseAlignAxisA=+Y  FollAlignAxisB=+Y  BaseAlignAxisB=+Z  RotationSequenceAxes=BaseAxes  RotationSequence=XYZ  RotationSequenceAngles=[0, -1, 0]  RotationSequenceAnglesUnits=rad  RotationMatrix=[0 0 -1;0 -1 0;-1 0 0]
  ReferenceFrame : sm_lib/Frames and Transforms/Reference Frame
  F : PMIOPort  Side=Left
  F1 : PMIOPort  Port=2  Side=Left
  connections:
  Inertia/RConn1 -- InertiaOriginTransform1/LConn1 -- InertiaOriginTransform/RConn1
  ReferenceFrame/RConn1 -- InertiaOriginTransform/LConn1 -- F/RConn1
  F1/RConn1 -- InertiaOriginTransform1/RConn1

== system variable_stiffness_Based_Position/SimscapeModelwithContactModel1/Rot_1_RIGID ==
  ReferenceFrame : sm_lib/Frames and Transforms/Reference Frame
  Solid : sm_lib/Body Elements/Solid  InertiaType=Custom  Mass=smiData.Solid(2).mass  MassUnits=kg  CenterOfMass=smiData.Solid(2).CoM  CenterOfMassUnits=mm  MomentsOfInertia=smiData.Solid(2).MoI  MomentsOfInertiaUnits=kg*mm^2  ProductsOfInertia=smiData.Solid(2).PoI  ProductsOfInertiaUnits=kg*mm^2  BasedOnType=Density  Density=1000  DensityUnits=kg/m^3  DoExposeReferenceFrame=on  SerializedFrames=<Frames/>  GraphicType=FromGeometry  MarkerShape=Sphere  MarkerSize=10  GraphicVisPropType=SimpleVisualProperties  GraphicDiffuseColor=smiData.Solid(2).color  GraphicSpecularColor=[0.5 0.5 0.5 1.0]  GraphicAmbientColor=[0.15 0.15 0.15 1.0]  GraphicEmissiveColor=[0.0 0.0 0.0 1.0]  GraphicShininess=75  GraphicOpacity=smiData.Solid(2).opacity  GeometryShape=FromFile  RectangleSize=[1 1]  RectangleSizeUnits=m  BrickDimensions=[1 1 1]  BrickDimensionUnits=m  CylinderRadius=1  CylinderRadiusUnits=m  CylinderLength=1  CylinderLengthUnits=m  SphereRadius=1  SphereRadiusUnits=m  EllipsoidRadii=[1 1 1]  EllipsoidRadiiUnits=m  ExtrusionCrossSection=[1 1; -1 1; -1 -1; 1 -1]  ExtrusionCrossSectionUnits=m  ExtrusionLength=1  ExtrusionLengthUnits=m  PolygonNumSides=3  PolygonOuterRadius=1  PolygonOuterRadiusUnits=m  ExtGeomFileType=STEP  ExtGeomFileName=Rot_默认_sldprt.STEP  ExtGeomFileUnits=m  RevolutionCrossSection=[1 1; 1 -1; 2 -1; 2 1]  RevolutionCrossSectionUnits=m  RevolutionExtent=Full  RevolutionAngle=180  RevolutionAngleUnits=deg
  Transform1 : sm_lib/Frames and Transforms/Rigid Transform  TranslationMethod=StandardAxis  TranslationStandardOffset=0  TranslationLengthUnit=mm  TranslationStandardAxis=+Z  TranslationCartesianOffset=smiData.RigidTransform(8).translation  TranslationROffset=0  TranslationROffsetUnits=m  TranslationZOffset=0  TranslationZOffsetUnits=m  TranslationThetaOffset=0  TranslationThetaOffsetUnits=deg  RotationMethod=RotationSequence  RotationAngleUnits=rad  RotationStandardAxis=+Z  RotationAngle=smiData.RigidTransform(8).angle  RotationArbitraryAxis=smiData.RigidTransform(8).axis  FollAlignAxisA=+X  BaseAlignAxisA=+Y  FollAlignAxisB=+Y  BaseAlignAxisB=+Z  RotationSequenceAxes=FollowerAxes  RotationSequence=XYX  RotationSequenceAngles=[0 0 0]  RotationSequenceAnglesUnits=deg  RotationMatrix=[1 0 0; 0 -1 0; 0 0 -1]
  Transform8 : sm_lib/Frames and Transforms/Rigid Transform  TranslationMethod=Cartesian  TranslationStandardOffset=0  TranslationLengthUnit=mm  TranslationStandardAxis=+Z  TranslationCartesianOffset=[0 0 -330]  TranslationROffset=0  TranslationROffsetUnits=m  TranslationZOffset=0  TranslationZOffsetUnits=m  TranslationThetaOffset=0  TranslationThetaOffsetUnits=deg  RotationMethod=RotationSequence  RotationAngleUnits=rad  RotationStandardAxis=+Z  RotationAngle=90  RotationArbitraryAxis=[0 1 0]  FollAlignAxisA=+X  BaseAlignAxisA=+Y  FollAlignAxisB=+Y  BaseAlignAxisB=+Z  RotationSequenceAxes=FollowerAxes  RotationSequence=XYX  RotationSequenceAngles=[0 0 0]  RotationSequenceAnglesUnits=deg  RotationMatrix=[1 0 0; 0 1 0; 0 0 1]
  F : PMIOPort  Side=Left
  endEff : PMIOPort  Port=2  Side=Right
  connections:
  endEff/RConn1 -- Transform1/RConn1
  ReferenceFrame/RConn1 -- Transform8/LConn1 -- F/RConn1
  Transform1/LConn1 -- Solid/RConn1 -- Transform8/RConn1

== system variable_stiffness_Based_Position/SimscapeModelwithContactModel1/Signal Builder ==
  Demux : Demux  Tag=STV Demux  Outputs=1
  FromWs : FromWorkspace  Tag=STV FromWs  VariableName=tuvar  SampleTime=0
      SigBuilderData=|
      | common.afterFinalStr = 'Extrapolate'
      | common.sampleTime = 0
      | dataSet.timeRange = [0 10]
      | dataSet.name = 'Group 1'
      | sbobj.Groups.Name = 'Group 1'
      | sbobj.Groups.Signals.Name = 'Signal 1'
      | sbobj.Groups.Signals.XData = [0 2 4 6 10]
      | sbobj.Groups.Signals.YData = [0 0 39.8 0 0]
  Signal 1 : Outport  Tag=STV Outport
  wires:
  Demux/1 -> Signal 1/1
  FromWs/1 -> Demux/1
